simulink library "lib_angle_mapper"  (R2023a)
settings: Solver=VariableStepAuto  StartTime=0.0  StopTime=10.0  RelTol=1e-3
settings Model: Creator=cav2ofo  LastModifiedBy=lenovo
settings OptimizationCC: ReuseModelBlockBuffer=off

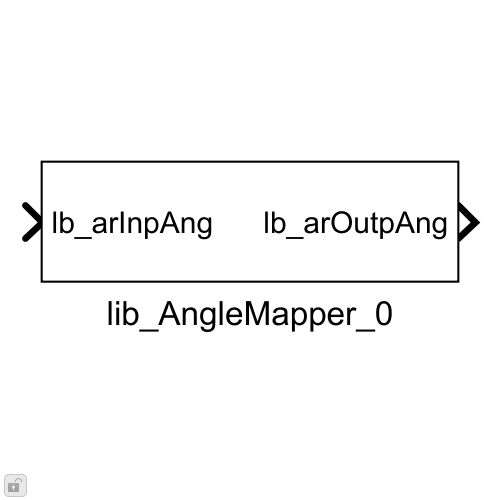
[thumbnail: Simulink's stored preview of the top-level diagram]
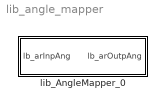
== system lib_angle_mapper ==
  lib_AngleMapper_0 : Subsystem  mask{lb_parSlctMappMode=[0,4pi] to [0,2pi], lb_parOutpDataType=Inherit: Inherit via back propagation}
      mask prompts: lb_parSlctMappMode "Select mapping mode:"; lb_parOutpDataType "Output data type:"
      mask init:
      | switch lb_parSlctMappMode
      |     
      |     case '[0,4pi] to [0,2pi]'
      |         lb_parSlctMappModeNum = 1;
      |         
      |     case '[-2pi,2pi] to [0,2pi]'
      |         lb_parSlctMappModeNum = 2;
      |         
      | end
      mask TypeOptions lb_parSlctMappMode: [0,4pi] to [0,2pi] | [-2pi,2pi] to [0,2pi]
      mask DialogControl DescGroupVar Prompt: VHIT control library
      mask DialogControl DescTextVar Prompt: Mapper for angles in radiant
      mask DialogControl ParameterGroupVar Prompt: Parameter
      mask DialogControl Container3 Prompt: Data type

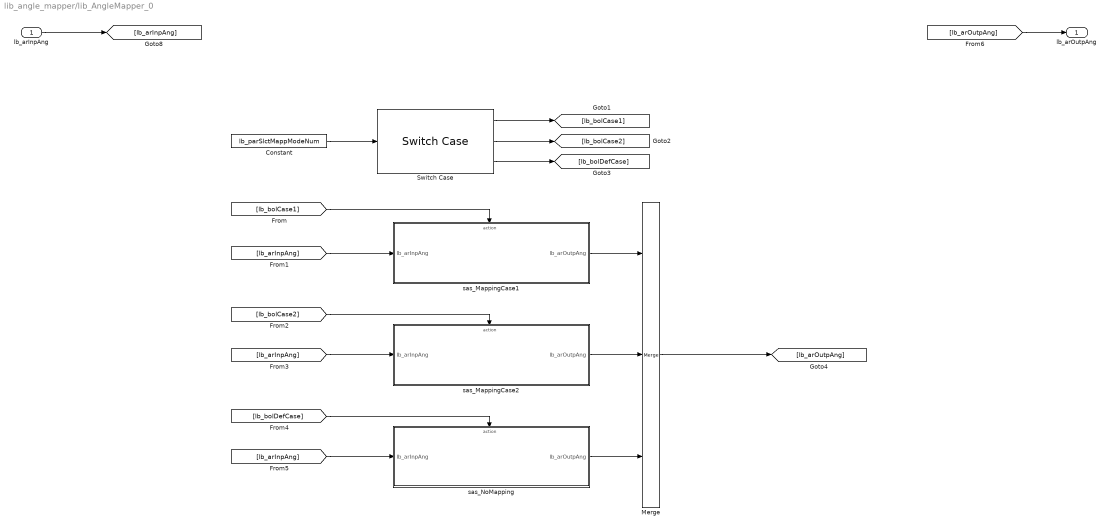
== system lib_angle_mapper/lib_AngleMapper_0 ==
  lb_arInpAng : Inport
  Constant : Constant  Value=lb_parSlctMappModeNum  OutDataTypeStr=uint8
  Merge : Merge  Inputs=3
  Switch Case : SwitchCase  CaseConditions={1,2}
  sas_MappingCase1 : Subsystem  TreatAsAtomicUnit=on
  sas_MappingCase2 : Subsystem  TreatAsAtomicUnit=on
  sas_NoMapping : Subsystem  TreatAsAtomicUnit=on
  lb_arOutpAng : Outport
  wires:
  Constant/1 -> Switch Case/1
  lb_arInpAng/1 -> [lb_arInpAng]
  Switch Case/1 -> [lb_bolCase1]
  Switch Case/2 -> [lb_bolCase2]
  Switch Case/3 -> [lb_bolDefCase]
  [lb_bolCase1] -> sas_MappingCase1/Action
  [lb_arInpAng] -> sas_MappingCase1/1(lb_arInpAng)
  [lb_bolCase2] -> sas_MappingCase2/Action
  [lb_arInpAng] -> sas_MappingCase2/1(lb_arInpAng)
  [lb_bolDefCase] -> sas_NoMapping/Action
  [lb_arInpAng] -> sas_NoMapping/1(lb_arInpAng)
  sas_MappingCase1/1(lb_arOutpAng) -> Merge/1
  sas_MappingCase2/1(lb_arOutpAng) -> Merge/2
  sas_NoMapping/1(lb_arOutpAng) -> Merge/3
  [lb_arOutpAng] -> lb_arOutpAng/1
  Merge/1 -> [lb_arOutpAng]

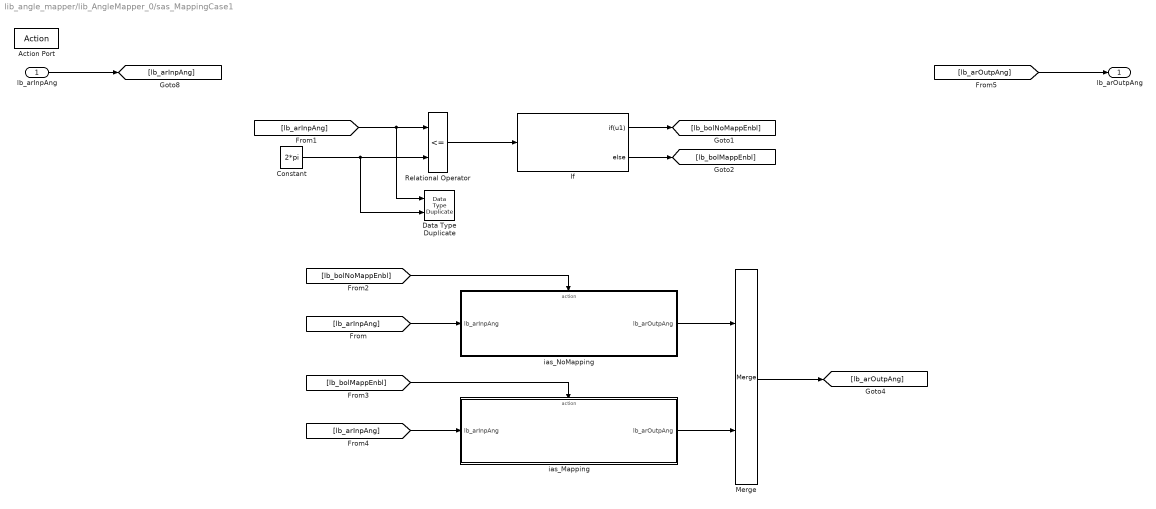
== system lib_angle_mapper/lib_AngleMapper_0/sas_MappingCase1 ==
  lb_arInpAng : Inport
  Action Port : ActionPort
  Constant : Constant  Value=2*pi  OutDataTypeStr=Inherit: Inherit via back propagation
  Data Type Duplicate : DataTypeDuplicate
  If : If  IfExpression=u1
  Merge : Merge
  Relational Operator : RelationalOperator  Operator=<=  OutDataTypeStr=boolean  RndMeth=Simplest  InputSameDT=off
  ias_Mapping : Subsystem  TreatAsAtomicUnit=on
  ias_NoMapping : Subsystem  TreatAsAtomicUnit=on
  lb_arOutpAng : Outport
  wires:
  Constant/1 -> Data Type Duplicate/2, Relational Operator/2
  [lb_arOutpAng] -> lb_arOutpAng/1
  Relational Operator/1 -> If/1
  lb_arInpAng/1 -> [lb_arInpAng]
  [lb_arInpAng] -> ias_NoMapping/1(lb_arInpAng)
  [lb_arInpAng] -> Data Type Duplicate/1, Relational Operator/1
  If/1 -> [lb_bolNoMappEnbl]
  If/2 -> [lb_bolMappEnbl]
  [lb_bolNoMappEnbl] -> ias_NoMapping/Action
  [lb_bolMappEnbl] -> ias_Mapping/Action
  [lb_arInpAng] -> ias_Mapping/1(lb_arInpAng)
  ias_NoMapping/1(lb_arOutpAng) -> Merge/1
  ias_Mapping/1(lb_arOutpAng) -> Merge/2
  Merge/1 -> [lb_arOutpAng]

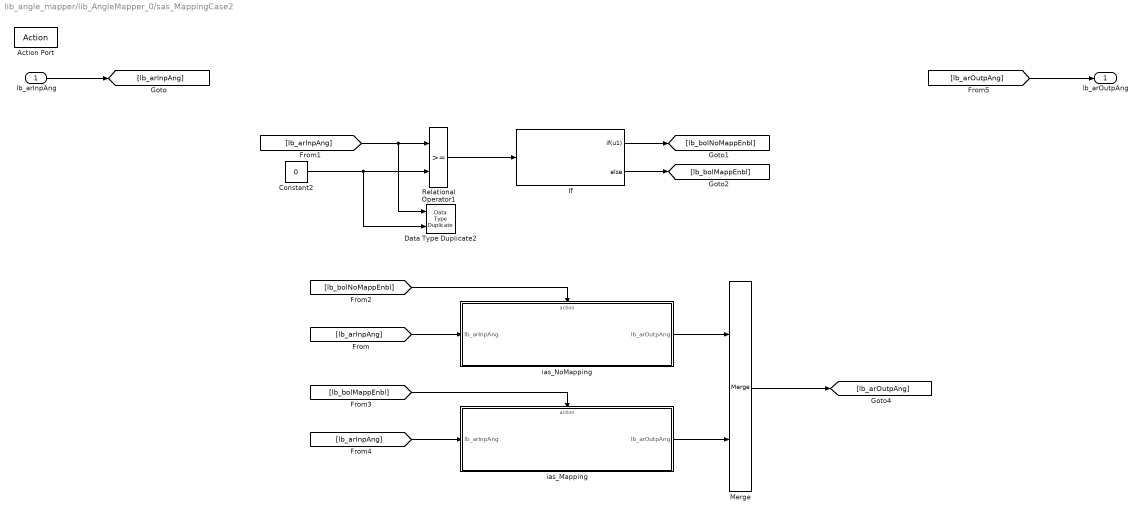
== system lib_angle_mapper/lib_AngleMapper_0/sas_MappingCase2 ==
  lb_arInpAng : Inport
  Action Port : ActionPort
  Constant2 : Constant  Value=0  OutDataTypeStr=Inherit: Inherit via back propagation
  Data Type Duplicate2 : DataTypeDuplicate
  If : If  IfExpression=u1
  Merge : Merge
  Relational Operator1 : RelationalOperator  OutDataTypeStr=boolean  RndMeth=Simplest  InputSameDT=off
  ias_Mapping : Subsystem  TreatAsAtomicUnit=on
  ias_NoMapping : Subsystem  TreatAsAtomicUnit=on
  lb_arOutpAng : Outport
  wires:
  [lb_arOutpAng] -> lb_arOutpAng/1
  [lb_bolNoMappEnbl] -> ias_NoMapping/Action
  ias_NoMapping/1(lb_arOutpAng) -> Merge/1
  [lb_bolMappEnbl] -> ias_Mapping/Action
  Relational Operator1/1 -> If/1
  If/2 -> [lb_bolMappEnbl]
  If/1 -> [lb_bolNoMappEnbl]
  [lb_arInpAng] -> Data Type Duplicate2/1, Relational Operator1/1
  [lb_arInpAng] -> ias_NoMapping/1(lb_arInpAng)
  [lb_arInpAng] -> ias_Mapping/1(lb_arInpAng)
  ias_Mapping/1(lb_arOutpAng) -> Merge/2
  Constant2/1 -> Data Type Duplicate2/2, Relational Operator1/2
  lb_arInpAng/1 -> [lb_arInpAng]
  Merge/1 -> [lb_arOutpAng]

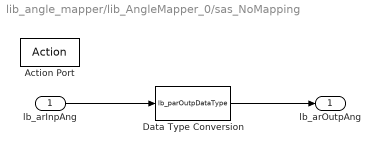
== system lib_angle_mapper/lib_AngleMapper_0/sas_NoMapping ==
  lb_arInpAng : Inport
  Action Port : ActionPort
  Data Type Conversion : DataTypeConversion  OutDataTypeStr=lb_parOutpDataType  SaturateOnIntegerOverflow=off  RndMeth=Floor
  lb_arOutpAng : Outport
  wires:
  lb_arInpAng/1 -> Data Type Conversion/1
  Data Type Conversion/1 -> lb_arOutpAng/1

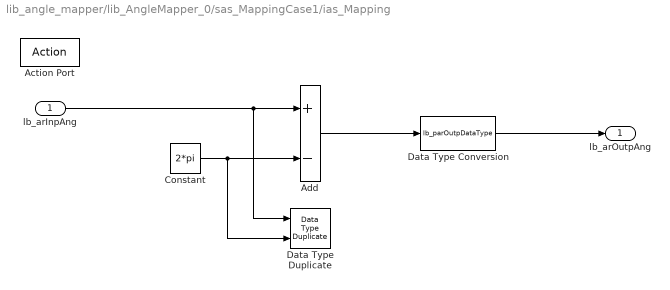
== system lib_angle_mapper/lib_AngleMapper_0/sas_MappingCase1/ias_Mapping ==
  lb_arInpAng : Inport
  Action Port : ActionPort
  Add : Sum  Inputs=+-  OutDataTypeStr=Inherit: Same as first input
  Constant : Constant  Value=2*pi  OutDataTypeStr=Inherit: Inherit via back propagation
  Data Type Duplicate : DataTypeDuplicate
  Data Type Conversion : DataTypeConversion  OutDataTypeStr=lb_parOutpDataType  SaturateOnIntegerOverflow=off  RndMeth=Floor
  lb_arOutpAng : Outport
  wires:
  lb_arInpAng/1 -> Data Type Duplicate/1, Add/1
  Constant/1 -> Data Type Duplicate/2, Add/2
  Add/1 -> Data Type Conversion/1
  Data Type Conversion/1 -> lb_arOutpAng/1

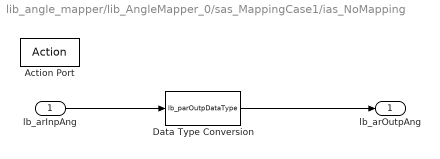
== system lib_angle_mapper/lib_AngleMapper_0/sas_MappingCase1/ias_NoMapping ==
  lb_arInpAng : Inport
  Action Port : ActionPort
  Data Type Conversion : DataTypeConversion  OutDataTypeStr=lb_parOutpDataType  SaturateOnIntegerOverflow=off  RndMeth=Floor
  lb_arOutpAng : Outport
  wires:
  lb_arInpAng/1 -> Data Type Conversion/1
  Data Type Conversion/1 -> lb_arOutpAng/1

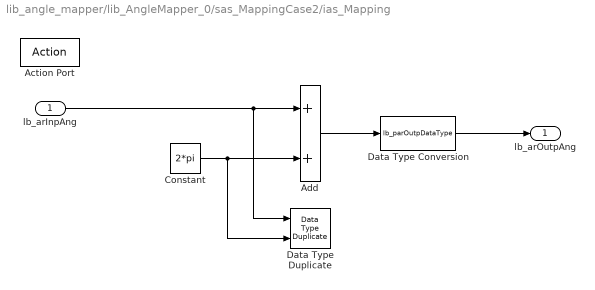
== system lib_angle_mapper/lib_AngleMapper_0/sas_MappingCase2/ias_Mapping ==
  lb_arInpAng : Inport
  Action Port : ActionPort
  Add : Sum  OutDataTypeStr=Inherit: Same as first input
  Constant : Constant  Value=2*pi  OutDataTypeStr=Inherit: Inherit via back propagation
  Data Type Duplicate : DataTypeDuplicate
  Data Type Conversion : DataTypeConversion  OutDataTypeStr=lb_parOutpDataType  SaturateOnIntegerOverflow=off  RndMeth=Floor
  lb_arOutpAng : Outport
  wires:
  lb_arInpAng/1 -> Data Type Duplicate/1, Add/1
  Constant/1 -> Data Type Duplicate/2, Add/2
  Add/1 -> Data Type Conversion/1
  Data Type Conversion/1 -> lb_arOutpAng/1

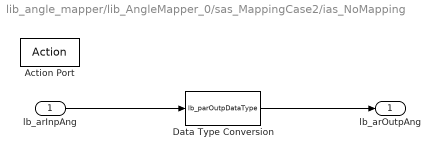
== system lib_angle_mapper/lib_AngleMapper_0/sas_MappingCase2/ias_NoMapping ==
  lb_arInpAng : Inport
  Action Port : ActionPort
  Data Type Conversion : DataTypeConversion  OutDataTypeStr=lb_parOutpDataType  SaturateOnIntegerOverflow=off  RndMeth=Floor
  lb_arOutpAng : Outport
  wires:
  lb_arInpAng/1 -> Data Type Conversion/1
  Data Type Conversion/1 -> lb_arOutpAng/1
